simulink model "simproj"  (R2024b)
settings: Solver=ode4  StartTime=0.0  StopTime=40  RelTol=1e-3
values from neighbouring files (symbols this model uses):
  Ka = 4.5    [missile.m]
  Kdc = 1.1    [missile.m]
  Ki = 14.3    [missile.m]
  Kr = -0.37    [missile.m]
  l_M0 = 80*d2r    (= 1.3962634016)    [missile.m]
  l_T0 = -2.5*d2r    (= -0.0436332312999)    [missile.m]
  V_T = 600    [missile.m]
  X_M0 = 2000    [missile.m]
  Z_M0 = 0    [missile.m]
libraries: simulink x1
settings Model: Creator=Kenny  LastModifiedBy=Kenny

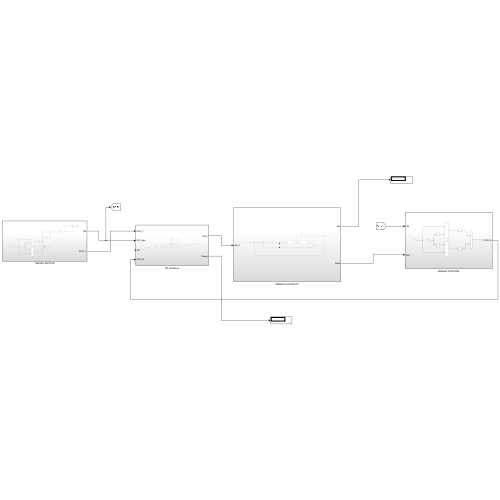
[thumbnail: Simulink's stored preview of the top-level diagram]
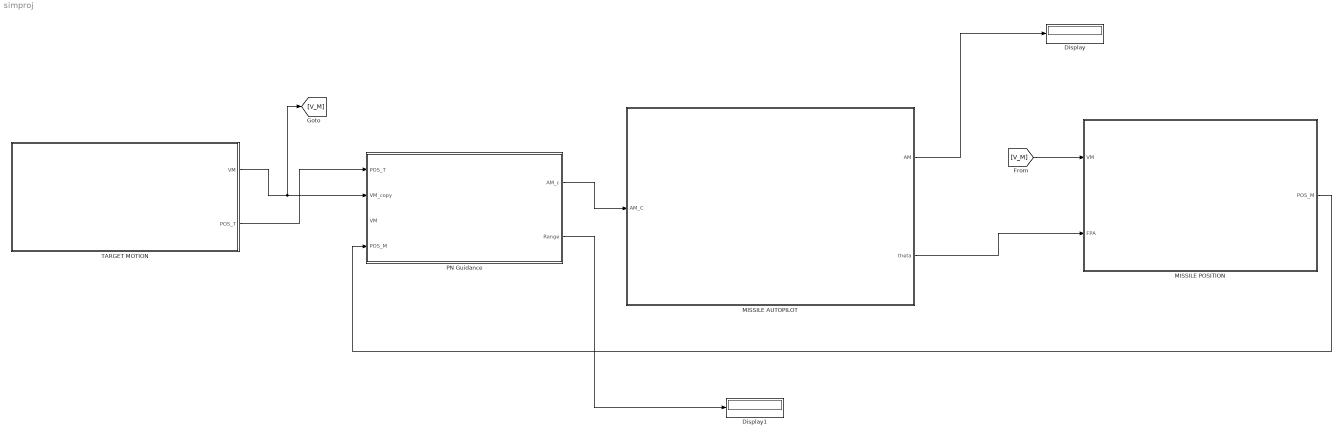
== system simproj ==
  Display : Display
  Display1 : Display
  MISSILE AUTOPILOT : Subsystem
  MISSILE POSITION : Subsystem
  PN Guidance : Subsystem
  TARGET MOTION : Subsystem
  wires:
  TARGET MOTION/2(POS_T) -> PN Guidance/1(POS_T)
  TARGET MOTION/1(VM) -> [V_M], PN Guidance/2(VM_copy)
  [V_M] -> MISSILE POSITION/1(VM)
  MISSILE POSITION/1(POS_M) -> PN Guidance/4(POS_M)
  PN Guidance/1(AM_c) -> MISSILE AUTOPILOT/1(AM_C)
  MISSILE AUTOPILOT/1(AM) -> Display/1
  MISSILE AUTOPILOT/2(theta) -> MISSILE POSITION/2(FPA)
  PN Guidance/2(Range) -> Display1/1

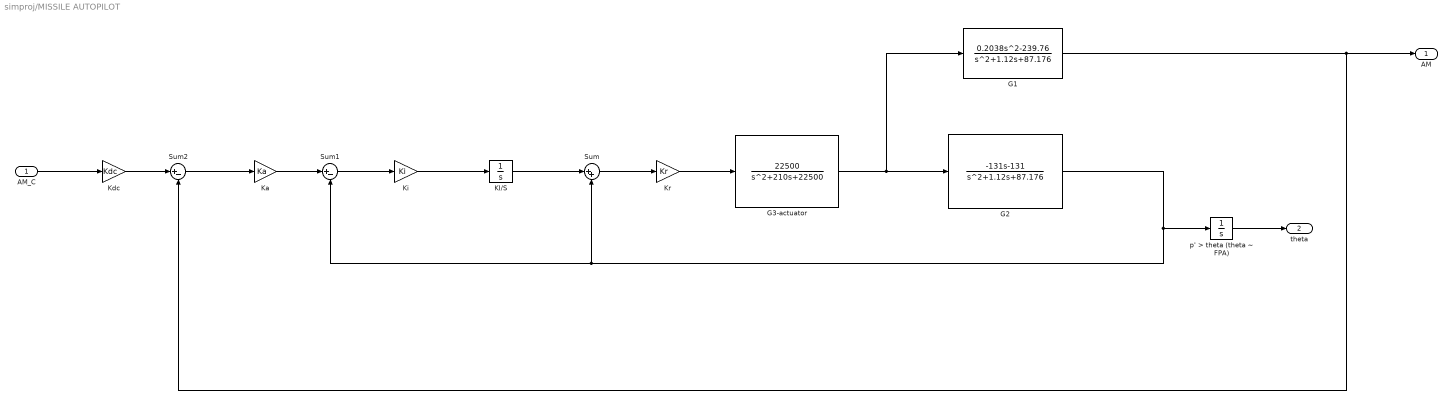
== system simproj/MISSILE AUTOPILOT ==
  AM_C : Inport
  G1 : TransferFcn  Numerator=[0.2038 0 -239.76]  Denominator=[1 1.12 87.176]
  G2 : TransferFcn  Numerator=[-131 -131]  Denominator=[1 1.12 87.176]
  G3-actuator : TransferFcn  Numerator=[22500]  Denominator=[1 210 22500]
  KI/S : Integrator
  Ka : Gain  Gain=Ka
  Kdc : Gain  Gain=Kdc
  Ki : Gain  Gain=Ki
  Kr : Gain  Gain=Kr
  Sum : Sum  Inputs=|++
  Sum1 : Sum  Inputs=|+-
  Sum2 : Sum  Inputs=|+-
  p' > theta (theta ~ FPA) : Integrator  InitialCondition=l_M0
  AM : Outport
  theta : Outport  Port=2
  wires:
  G1/1 -> AM/1, Sum2/2
  G3-actuator/1 -> G1/1, G2/1
  KI/S/1 -> Sum/1
  Sum/1 -> Kr/1
  Ka/1 -> Sum1/1
  G2/1 -> Sum1/2, Sum/2, p' > theta (theta ~ FPA)/1
  Ki/1 -> KI/S/1
  Sum2/1 -> Ka/1
  Kr/1 -> G3-actuator/1
  Sum1/1 -> Ki/1
  p' > theta (theta ~ FPA)/1 -> theta/1
  Kdc/1 -> Sum2/1
  AM_C/1 -> Kdc/1

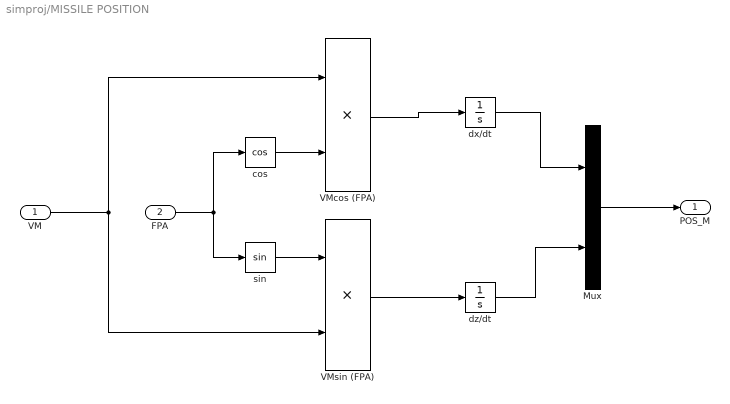
== system simproj/MISSILE POSITION ==
  VM : Inport
  FPA : Inport  Port=2
  Mux : Mux  Inputs=2
  VMcos (FPA) : Product
  VMsin (FPA) : Product
  cos : Trigonometry  Operator=cos
  dx/dt : Integrator  InitialCondition=X_M0
  dz/dt : Integrator  InitialCondition=Z_M0
  sin : Trigonometry
  POS_M : Outport
  wires:
  dx/dt/1 -> Mux/1
  cos/1 -> VMcos (FPA)/2
  Mux/1 -> POS_M/1
  dz/dt/1 -> Mux/2
  FPA/1 -> sin/1, cos/1
  VMsin (FPA)/1 -> dz/dt/1
  VM/1 -> VMsin (FPA)/2, VMcos (FPA)/1
  VMcos (FPA)/1 -> dx/dt/1
  sin/1 -> VMsin (FPA)/1

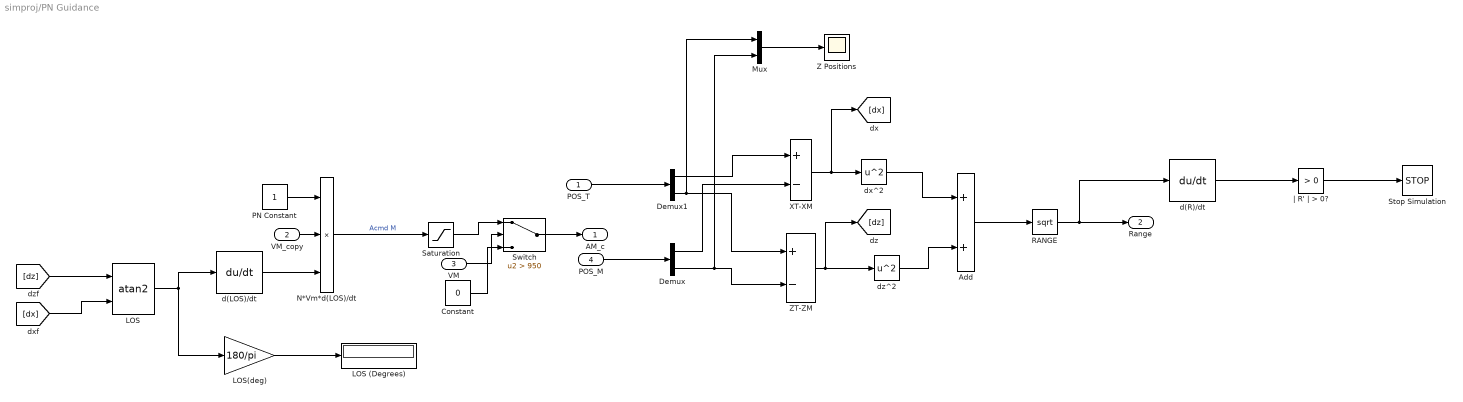
== system simproj/PN Guidance ==
  POS_T : Inport
  VM_copy : Inport  Port=2
  VM : Inport  Port=3
  POS_M : Inport  Port=4
  Add : Sum
  Constant : Constant  Value=0
  Demux : Demux  Outputs=2
  Demux1 : Demux  Outputs=2
  LOS : Trigonometry  Operator=atan2
  LOS (Degrees) : Display
  LOS(deg) : Gain  Gain=180/pi
  Mux : Mux  Inputs=2
  N*Vm*d(LOS)/dt : Product  Inputs=3
  PN Constant : Constant
  RANGE : Sqrt
  Saturation : Saturate  UpperLimit=0  LowerLimit=-0.1
  Stop Simulation : Stop
  Switch : Switch  Criteria=u2 > Threshold  Threshold=950  SaturateOnIntegerOverflow=off  InputSameDT=off
  XT-XM : Sum  Inputs=+-
  Z Positions : Scope
  ZT-ZM : Sum  Inputs=+-
  d(LOS)/dt : Derivative
  d(R)/dt : Derivative
  dx^2 : Math  Operator=square
  dz^2 : Math  Operator=square
  | R' | > 0? : simulink/Logic and Bit Operations/Compare To Zero  relop=>  OutDataTypeStr=boolean
  AM_c : Outport
  Range : Outport  Port=2
  wires:
  Saturation/1 -> Switch/1
  RANGE/1 -> Range/1, d(R)/dt/1
  LOS/1 -> d(LOS)/dt/1, LOS(deg)/1
  PN Constant/1 -> N*Vm*d(LOS)/dt/1
  d(LOS)/dt/1 -> N*Vm*d(LOS)/dt/3
  XT-XM/1 -> [dx], dx^2/1
  LOS(deg)/1 -> LOS (Degrees)/1
  POS_T/1 -> Demux1/1
  ZT-ZM/1 -> [dz], dz^2/1
  Demux/2 -> Mux/2, ZT-ZM/2
  Mux/1 -> Z Positions/1
  VM_copy/1 -> N*Vm*d(LOS)/dt/2
  [dx] -> LOS/2
  Switch/1 -> AM_c/1
  | R' | > 0?/1 -> Stop Simulation/1
  [dz] -> LOS/1
  N*Vm*d(LOS)/dt/1 -> Saturation/1  "Acmd M"
  Demux1/1 -> XT-XM/1
  Demux1/2 -> Mux/1, ZT-ZM/1
  VM/1 -> Switch/2
  d(R)/dt/1 -> | R' | > 0?/1
  Demux/1 -> XT-XM/2
  POS_M/1 -> Demux/1
  dx^2/1 -> Add/1
  Add/1 -> RANGE/1
  dz^2/1 -> Add/2
  Constant/1 -> Switch/3

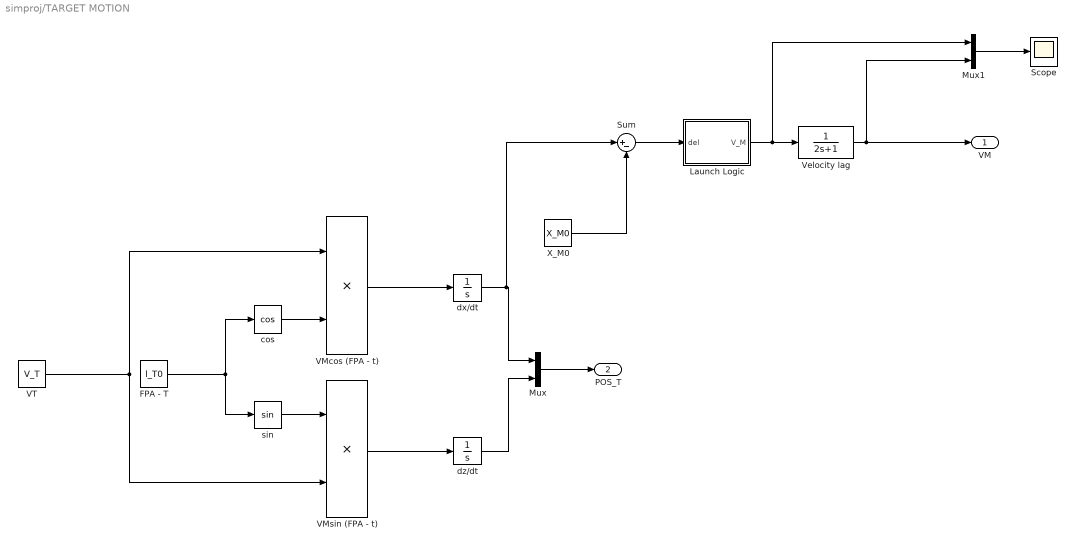
== system simproj/TARGET MOTION ==
  FPA - T : Constant  Value=l_T0
  Launch Logic : MATLAB Function  TreatAsAtomicUnit=on
  Mux : Mux  Inputs=2
  Mux1 : Mux  Inputs=2
  Scope : Scope
  Sum : Sum  Inputs=|+-
  VMcos (FPA - t) : Product
  VMsin (FPA - t) : Product
  VT : Constant  Value=V_T
  Velocity lag : TransferFcn  Denominator=[2 1]
  X_M0 : Constant  Value=X_M0
  cos : Trigonometry  Operator=cos
  dx/dt : Integrator  InitialCondition=V_T
  dz/dt : Integrator  InitialCondition=Z_M0
  sin : Trigonometry
  VM : Outport
  POS_T : Outport  Port=2
  wires:
  FPA - T/1 -> sin/1, cos/1
  X_M0/1 -> Sum/2
  Velocity lag/1 -> VM/1, Mux1/2
  sin/1 -> VMsin (FPA - t)/1
  VMsin (FPA - t)/1 -> dz/dt/1
  VT/1 -> VMsin (FPA - t)/2, VMcos (FPA - t)/1
  cos/1 -> VMcos (FPA - t)/2
  VMcos (FPA - t)/1 -> dx/dt/1
  Launch Logic/1(V_M) -> Mux1/1, Velocity lag/1
  dz/dt/1 -> Mux/2
  dx/dt/1 -> Sum/1, Mux/1
  Mux/1 -> POS_T/1
  Sum/1 -> Launch Logic/1(del)
  Mux1/1 -> Scope/1

== matlab function simproj/TARGET MOTION/Launch Logic ==
  settings: updateMethod=DISCRETE
  data: del input; V_M output
function V_M = fcn(del)
%#codegen

persistent f
persistent Vel

if isempty(f)
    f = 0;
end
if isempty(Vel)
    Vel = 0;
end

if f == 0 && del > -200
    f = 1;
    Vel = 1021; % missile speed
end

V_M = Vel;
